simulink model "pid_poles_alocation"  (R2023a)
settings: Solver=VariableStepAuto  StartTime=0.0  StopTime=10.0  RelTol=1e-3
values from neighbouring files (symbols this model uses):
  a = a1    (= 0.005)    [controle.m]
settings Model: Creator=omega  LastModifiedBy=omega

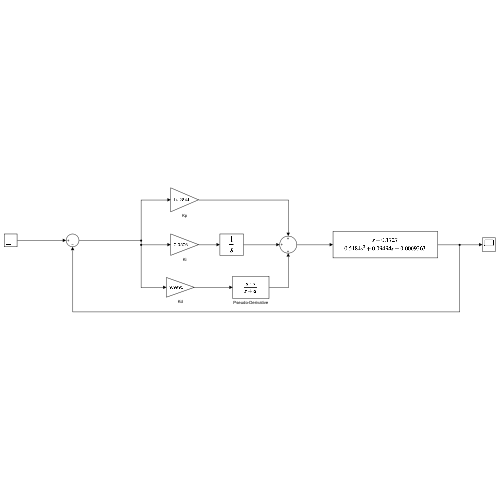
[thumbnail: Simulink's stored preview of the top-level diagram]
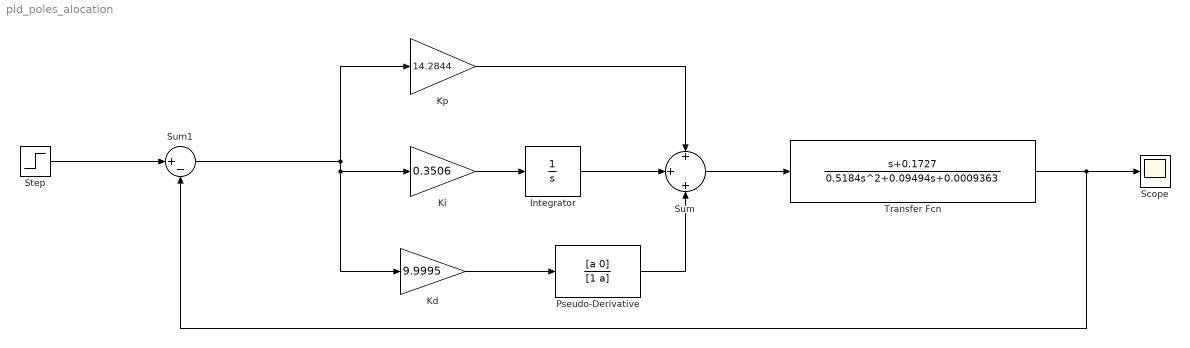
== system pid_poles_alocation ==
  Integrator : Integrator
  Kd : Gain  Gain=9.9995
  Ki : Gain  Gain=0.3506
  Kp : Gain  Gain=14.2844
  Pseudo-Derivative : TransferFcn  Numerator=[a 0]  Denominator=[1 a]
  Scope : Scope
  Step : Step  SampleTime=0
  Sum : Sum  Inputs=+||+||+
  Sum1 : Sum  Inputs=|+-
  Transfer Fcn : TransferFcn  Numerator=[1 0.1727]  Denominator=[0.5184 0.09494 0.0009363]
  wires:
  Kp/1 -> Sum/1
  Integrator/1 -> Sum/2
  Pseudo-Derivative/1 -> Sum/3
  Kd/1 -> Pseudo-Derivative/1
  Ki/1 -> Integrator/1
  Sum/1 -> Transfer Fcn/1
  Step/1 -> Sum1/1
  Sum1/1 -> Kd/1, Ki/1, Kp/1
  Transfer Fcn/1 -> Scope/1, Sum1/2
